simulink model "Five_state_LQR_simulation"  (R2020a)
settings: Solver=ode1  StartTime=0.0  StopTime=20  FixedStep=0.002  RelTol=1e-3  EnableMultiTasking=on
PostLoadFcn:
  | qc_set_target_type(getConfigSet(bdroot, 'QUARC Default Target Configuration'));
values from neighbouring files (symbols this model uses):
  F = [K(1,1),K(1,3);K(2,1),K(2,3)]    [Five_state_LQR_init.m]
undefined symbols (not defined in the file or in its folder): A_hat, B_hat, K
settings Model: SimulationMode=external  ExtModeTrigDuration=60000  Creator=Rchan  LastModifiedBy=olav_
settings SolverCC: PositivePriorityOrder=on
settings DataIOCC: SaveFormat=Array  SignalLoggingSaveFormat=ModelDataLogs  ReturnWorkspaceOutputs=off
settings OptimizationCC: ExpressionDepthLimit=2147483647  InitFltsAndDblsToZero=on  LifeSpan=inf
settings DebuggingCC: SaveWithParameterizedLinksMsg=none  UnderspecifiedInitializationDetection=Classic  MergeDetectMultiDrivingBlocksExec=none  SolverPrmCheckMsg=warning  MultiTaskDSMMsg=warning  MultiTaskCondExecSysMsg=none  FcnCallInpInsideContextMsg=warning  AllowSymbolicDim=off  StateNameClashWarn=warning  SFUnexpectedBacktrackingDiag=warning  SFNoUnconditionalDefaultTransitionDiag=warning  SFExecutionAtInitializationDiag=none  ArithmeticOperatorsInVariantConditions=warning
settings HardwareCC: ProdBitPerPointer=32  ProdBitPerSizeT=32  ProdBitPerPtrDiffT=32  ProdLargestAtomicFloat=None  ProdIntDivRoundTo=Undefined  ProdEndianess=Unspecified  ProdWordSize=32  ProdHWDeviceType=32-bit Generic
settings ModelReferenceCC: PropagateSignalLabelsOutOfModel=off
settings SFSimCC: SimUseLocalCustomCode=off  CustomCodeUndefinedFunction=UseInterfaceOnly
settings RTWCC: Description=QUARC Win64 Target  SystemTargetFile=quarc_win64.tlc  TemplateMakefile=quarc_default_tmf  RTWUseLocalCustomCode=off
settings CodeAppCC: StateflowObjectComments=on
settings STFCustomTargetCC: TargetPreCompLibLocation=C:\PROGRA~3\QUARC\lib\2015b\win64\release  ConcurrentExecutionCompliant=on  CPPClassGenCompliant=on  GRTInterface=on  SystemTargetFile=quarc_win64.tlc
settings GRTTargetCC: TargetPreCompLibLocation=C:\PROGRA~3\QUARC\lib\2015b\win64\release  TargetLangStandard=C89/C90 (ANSI)  ParMdlRefBuildCompliant=off  CompOptLevelCompliant=off  CombineOutputUpdateFcns=off  MatFileLogging=off  GRTInterface=on  UseToolchainInfoCompliant=off  ExtMode=on  ExtModeMexFile=quarc_comm
settings ConfigComp: CovMetricSettings=dw  CovHtmlReporting=on  CovSaveCumulativeToWorkspaceVar=on  CovSaveSingleToWorkspaceVar=on  CovExternalEMLEnable=off  CovSFcnEnable=off

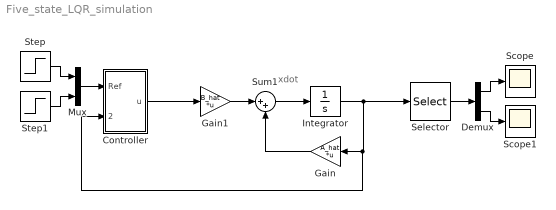
== system Five_state_LQR_simulation ==
  note: xdot
  Controller : Subsystem
  Demux : Demux  Outputs=2
  Gain : Gain  Gain=A_hat  Multiplication=Matrix(K*u)
  Gain1 : Gain  Gain=B_hat  Multiplication=Matrix(K*u)
  Integrator : Integrator
  Mux : Mux  Inputs=2
  Scope : Scope
  Scope1 : Scope
  Selector : Selector  InputPortWidth=6  IndexOptions=Index vector (dialog)  Indices=[1 4]  OutputSizes=1
  Step : Step  Time=0  After=0  SampleTime=0
  Step1 : Step  After=5  SampleTime=0
  Sum1 : Sum  Inputs=|++
  wires:
  Gain1/1 -> Sum1/1
  Sum1/1 -> Integrator/1
  Gain/1 -> Sum1/2
  Integrator/1 -> Selector/1, Controller/2(States), Gain/1
  Controller/1(u) -> Gain1/1
  Selector/1 -> Demux/1
  Mux/1 -> Controller/1(Ref)
  Step1/1 -> Mux/2
  Step/1 -> Mux/1
  Demux/1 -> Scope/1
  Demux/2 -> Scope1/1

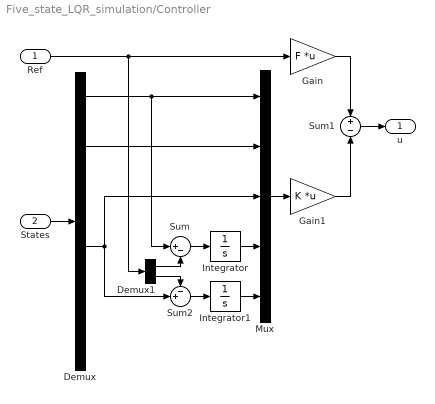
== system Five_state_LQR_simulation/Controller ==
  Ref : Inport
  States : Inport  Port=2
  Demux : Demux  Outputs=6
  Demux1 : Demux  Outputs=2
  Gain : Gain  Gain=F  Multiplication=Matrix(K*u)
  Gain1 : Gain  Gain=K  Multiplication=Matrix(K*u)
  Integrator : Integrator
  Integrator1 : Integrator
  Mux : Mux  Inputs=5
  Sum : Sum  Inputs=|+-
  Sum1 : Sum  Inputs=+|-
  Sum2 : Sum  Inputs=-+|
  u : Outport
  wires:
  Gain/1 -> Sum1/1
  Sum1/1 -> u/1
  Ref/1 -> Gain/1, Demux1/1
  Gain1/1 -> Sum1/2
  Sum/1 -> Integrator/1
  States/1 -> Demux/1
  Demux/1 -> Mux/1, Sum/1
  Demux/2 -> Mux/2
  Demux/4 -> Sum2/2, Mux/3
  Demux1/1 -> Sum/2
  Integrator/1 -> Mux/4
  Mux/1 -> Gain1/1
  Integrator1/1 -> Mux/5
  Sum2/1 -> Integrator1/1
  Demux1/2 -> Sum2/1
